simulink model "ARDroneWPTracking"  (R2018b)
settings: Solver=ode1  StartTime=0.0  StopTime=inf  FixedStep=sampleTime  RelTol=1e-3  EnableMultiTasking=on
undefined symbols (not defined in the file): Gxd_A_obs, Gxd_B_obs, Gxd_C_obs, Gyawd_A_obs, Gyawd_B_obs, Gyawd_C_obs, Gyd_A_obs, Gyd_B_obs, Gyd_C_obs, Gzd_A_obs, Gzd_B_obs, Gzd_C_obs, K0_X, K0_Y, K0_yaw, K0_Z, K_X, K_Y, K_yaw, K_Z, KGe_X, KGe_Y, KGe_yaw, KGe_Z, sampleTime, Standard_Devices, t_samp, UDP_Protocol, waypoints
libraries: sldrtlib x2, rtwinlib x1
CloseFcn:
  | rtwprivate ssgencode ModelCloseRequest Good_NL_model
settings Model: SimulationMode=external  ExtModeTrigDuration=100000  Creator=Paul  LastModifiedBy=Henrique
settings DataIOCC: LimitDataPoints=on  SaveFormat=Array  SignalLoggingSaveFormat=ModelDataLogs  TimeSaveName=time
settings OptimizationCC: ExpressionDepthLimit=2147483647  InitFltsAndDblsToZero=on
settings DebuggingCC: UnderspecifiedInitializationDetection=Classic  MergeDetectMultiDrivingBlocksExec=none  SolverPrmCheckMsg=warning  FcnCallInpInsideContextMsg=warning  StateNameClashWarn=warning  SFUnexpectedBacktrackingDiag=warning  SFNoUnconditionalDefaultTransitionDiag=warning  SFExecutionAtInitializationDiag=none
settings ModelReferenceCC: PropagateSignalLabelsOutOfModel=off
settings SFSimCC: SimUseLocalCustomCode=off
settings RTWCC: SystemTargetFile=sldrt.tlc  TemplateMakefile=sldrt.tmf  Description=Simulink Desktop Real-Time  RTWUseLocalCustomCode=off  RTWCompilerOptimization=on
settings CodeAppCC: MaxIdLength=95  StateflowObjectComments=on
settings SimulinkDesktopRealTimeCC: TargetPreCompLibLocation=D:\Programas\MATLAB 2018b\toolbox\sldrt\lib\win64  TargetLangStandard=C89/C90 (ANSI)  SupportVariableSizeSignals=off  PreserveStateflowLocalDataDimensions=off
settings ConfigComp: CovMetricSettings=dw  CovHtmlReporting=on  CovSaveCumulativeToWorkspaceVar=on  CovSaveSingleToWorkspaceVar=on  CovExternalEMLEnable=off

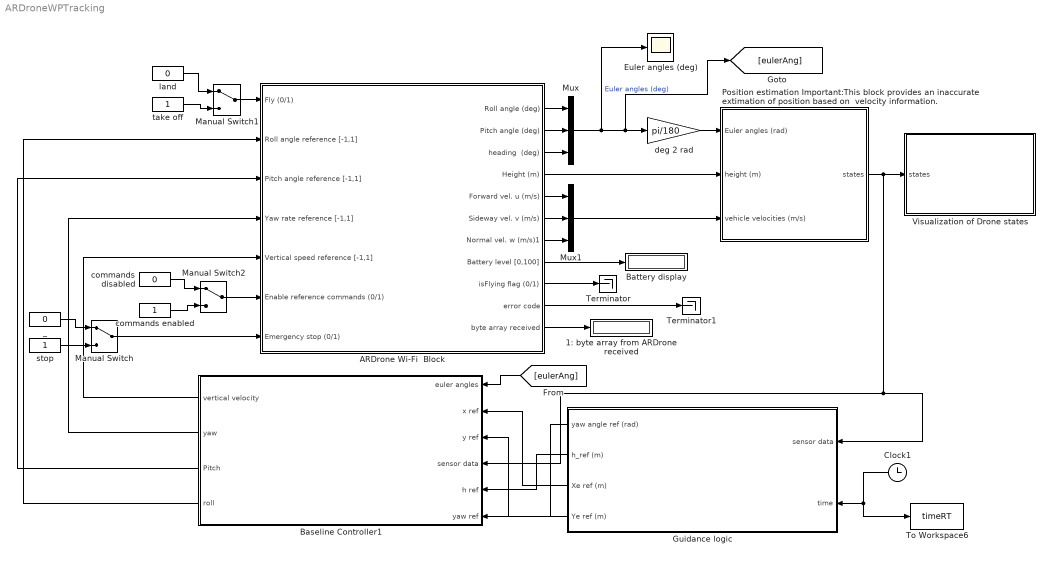
== system ARDroneWPTracking ==
  "1: byte array from ARDrone received " : Display
  ARDrone Wi-Fi  Block : Subsystem  AncestorBlock="ARBlocks/ARDrone Wi-Fi  Block"
  Baseline Controller1 : Subsystem  AncestorBlock=ARBlocks/Baseline Controller
  Battery display : Display
  Clock1 : Clock
  Euler angles (deg) : Scope
  Guidance logic : Subsystem  AncestorBlock=ARBlocks/Guidance logic
  Manual Switch : ManualSwitch
  Manual Switch1 : ManualSwitch
  Manual Switch2 : ManualSwitch
  Mux : Mux  Inputs=3
  Mux1 : Mux  Inputs=3
  "Position estimation Important:This block provides an inaccurate extimation of position based on  velocity information. " : Subsystem  AncestorBlock=|
      | ARBlocks/Position estimation
      | Important:This block provides an 
      | inaccurate extimation of position 
      | based on  velocity information.
  Terminator : Terminator
  Terminator1 : Terminator
  To Workspace6 : ToWorkspace  VariableName=timeRT  SampleTime=sampleTime
  Visualization of Drone states : Subsystem
  _ : Constant  Value=0
  commands disabled : Constant  Value=0
  commands enabled : Constant
  deg 2 rad : Gain  Gain=pi/180
  land : Constant  Value=0
  stop : Constant
  take off : Constant
  wires:
  _/1 -> Manual Switch/1
  stop/1 -> Manual Switch/2
  land/1 -> Manual Switch1/1
  take off/1 -> Manual Switch1/2
  commands disabled/1 -> Manual Switch2/1
  commands enabled/1 -> Manual Switch2/2
  Manual Switch1/1 -> ARDrone Wi-Fi  Block/1(Fly (0/1))
  Manual Switch2/1 -> ARDrone Wi-Fi  Block/6(Enable reference commands (0/1))
  Manual Switch/1 -> ARDrone Wi-Fi  Block/7(Emergency stop (0/1))
  ARDrone Wi-Fi  Block/1(Roll angle (deg)) -> Mux/1
  ARDrone Wi-Fi  Block/2(Pitch angle (deg)) -> Mux/2
  ARDrone Wi-Fi  Block/5(Forward vel. u (m/s)) -> Mux1/1
  ARDrone Wi-Fi  Block/6(Sideway vel. v (m/s)) -> Mux1/2
  ARDrone Wi-Fi  Block/7(Normal vel. w (m/s)1) -> Mux1/3
  Mux/1 -> Euler angles (deg)/1, [eulerAng], deg 2 rad/1  "Euler angles (deg)"
  ARDrone Wi-Fi  Block/8(Battery level [0,100]) -> Battery display/1
  "Position estimation Important:This block provides an inaccurate extimation of position based on  velocity information. "/1(states) -> Baseline Controller1/4(sensor data), Guidance logic/1(sensor data), Visualization of Drone states/1(states)
  deg 2 rad/1 -> "Position estimation Important:This block provides an inaccurate extimation of position based on  velocity information. "/1(Euler angles (rad))
  ARDrone Wi-Fi  Block/4(Height (m)) -> "Position estimation Important:This block provides an inaccurate extimation of position based on  velocity information. "/2(height (m))
  Mux1/1 -> "Position estimation Important:This block provides an inaccurate extimation of position based on  velocity information. "/3(vehicle velocities (m/s))
  Clock1/1 -> To Workspace6/1, Guidance logic/2(time)
  ARDrone Wi-Fi  Block/3(heading  (deg)) -> Mux/3
  Guidance logic/2(h_ref (m)) -> Baseline Controller1/5(h ref)
  Guidance logic/4(Ye ref (m)) -> Baseline Controller1/3(y ref)
  Guidance logic/1(yaw angle ref (rad)) -> Baseline Controller1/6(yaw ref)
  ARDrone Wi-Fi  Block/9(isFlying flag (0/1)) -> Terminator/1
  ARDrone Wi-Fi  Block/10(error code) -> Terminator1/1
  ARDrone Wi-Fi  Block/11(byte array received) -> "1: byte array from ARDrone received "/1
  Guidance logic/3(Xe ref (m)) -> Baseline Controller1/2(x ref)
  [eulerAng] -> Baseline Controller1/1(euler angles)
  Baseline Controller1/1("vertical velocity ") -> ARDrone Wi-Fi  Block/5(Vertical speed reference [-1,1])
  Baseline Controller1/2("yaw ") -> ARDrone Wi-Fi  Block/4(Yaw rate reference [-1,1])
  Baseline Controller1/3("Pitch ") -> ARDrone Wi-Fi  Block/3(Pitch angle reference [-1,1])
  Baseline Controller1/4("roll ") -> ARDrone Wi-Fi  Block/2(Roll angle reference [-1,1])

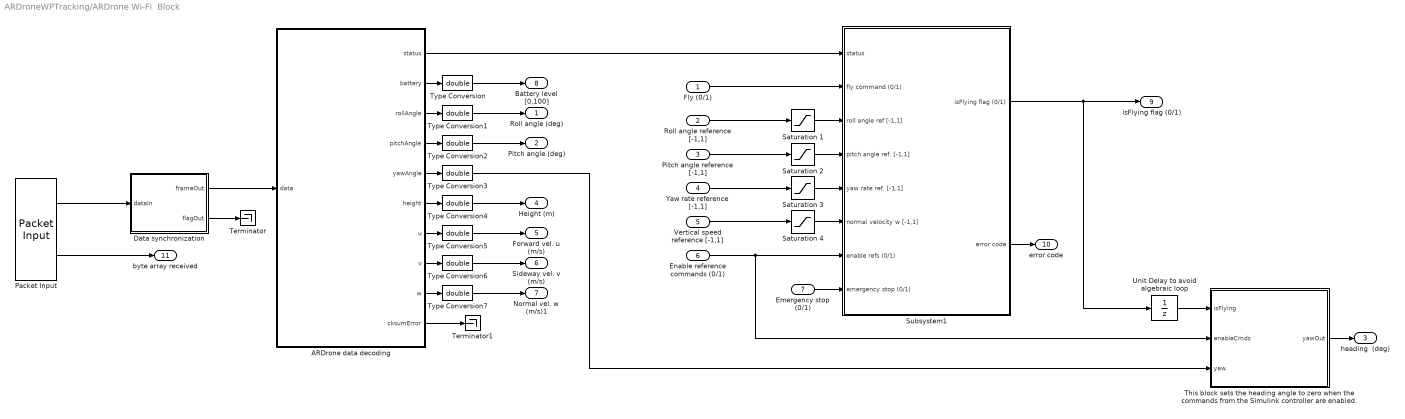
== system ARDroneWPTracking/ARDrone Wi-Fi  Block ==
  Fly (0/1) : Inport
  Roll angle reference [-1,1] : Inport  Port=2
  Pitch angle reference [-1,1] : Inport  Port=3
  Yaw rate reference [-1,1] : Inport  Port=4
  Vertical speed reference [-1,1] : Inport  Port=5
  Enable reference commands (0/1) : Inport  Port=6
  Emergency stop (0/1) : Inport  Port=7
  ARDrone data decoding : MATLAB Function  TreatAsAtomicUnit=on
  "Data synchronization " : MATLAB Function  TreatAsAtomicUnit=on
  Packet Input : sldrtlib/Packet Input  SampleTime=sampleTime  MaxMissedTicks=1  ShowMissedTicks=off  YieldWhenWaiting=off  DrvName=Standard_Devices/UDP_Protocol  DrvAddress=5554  DrvOptions=[3232235777 5554]  PacketSize=500  DataTypes='500*uint8'  ShowReady=on  ShowError=off  PacketID=1  ByteOrder=1  ShowTimestamp=off
      settings: AttributesFormatString=Standard Devices\nUDP Protocol [15B2h]  SourceProductName=Simulink Desktop Real-Time
  Saturation {1..4} (4 alike) : Saturate  UpperLimit=1  LowerLimit=-1
  Subsystem1 : Subsystem
  Terminator : Terminator
  Terminator1 : Terminator
  "This block sets the heading angle to zero when the commands from the Simulink controller are enabled. " : MATLAB Function  TreatAsAtomicUnit=on
  Type Conversion{,1..7} (8 alike) : DataTypeConversion  OutDataTypeStr=double
  Unit Delay to avoid algebraic loop : UnitDelay  SampleTime=-1
  Roll angle (deg) : Outport
  Pitch angle (deg) : Outport  Port=2
  heading  (deg) : Outport  Port=3
  Height (m) : Outport  Port=4
  Forward vel. u (m/s) : Outport  Port=5
  Sideway vel. v (m/s) : Outport  Port=6
  Normal vel. w (m/s)1 : Outport  Port=7
  Battery level [0,100] : Outport  Port=8
  isFlying flag (0/1) : Outport  Port=9
  error code : Outport  Port=10
  byte array received : Outport  Port=11
  wires:
  Unit Delay to avoid algebraic loop/1 -> "This block sets the heading angle to zero when the commands from the Simulink controller are enabled. "/1(isFlying)
  "Data synchronization "/2(flagOut) -> Terminator/1
  Saturation 4/1 -> Subsystem1/6(normal velocity w [-1,1])
  Saturation 3/1 -> Subsystem1/5(yaw rate ref. [-1,1])
  Saturation 2/1 -> Subsystem1/4(pitch angle ref. [-1,1])
  Saturation 1/1 -> Subsystem1/3(roll angle ref [-1,1])
  Fly (0/1)/1 -> Subsystem1/2(fly command (0/1))
  "This block sets the heading angle to zero when the commands from the Simulink controller are enabled. "/1(yawOut) -> heading  (deg)/1
  Type Conversion3/1 -> "This block sets the heading angle to zero when the commands from the Simulink controller are enabled. "/3(yaw)
  Type Conversion7/1 -> Normal vel. w (m/s)1/1
  Type Conversion6/1 -> Sideway vel. v (m/s)/1
  Type Conversion5/1 -> Forward vel. u (m/s)/1
  Type Conversion4/1 -> Height (m)/1
  Type Conversion2/1 -> Pitch angle (deg)/1
  Type Conversion1/1 -> Roll angle (deg)/1
  Type Conversion/1 -> Battery level [0,100]/1
  ARDrone data decoding/10(cksumError) -> Terminator1/1
  Subsystem1/2(error code) -> error code/1
  Subsystem1/1(isFlying flag (0/1)) -> Unit Delay to avoid algebraic loop/1, isFlying flag (0/1)/1
  Emergency stop (0/1)/1 -> Subsystem1/8(emergency stop (0/1))
  Enable reference commands (0/1)/1 -> Subsystem1/7(enable refs (0/1)), "This block sets the heading angle to zero when the commands from the Simulink controller are enabled. "/2(enableCmds)
  Vertical speed reference [-1,1]/1 -> Saturation 4/1
  Yaw rate reference [-1,1]/1 -> Saturation 3/1
  Pitch angle reference [-1,1]/1 -> Saturation 2/1
  Roll angle reference [-1,1]/1 -> Saturation 1/1
  ARDrone data decoding/1(status) -> Subsystem1/1(status)
  Packet Input/2 -> byte array received/1
  ARDrone data decoding/9(w) -> Type Conversion7/1
  ARDrone data decoding/8(v) -> Type Conversion6/1
  ARDrone data decoding/7(u) -> Type Conversion5/1
  ARDrone data decoding/4(pitchAngle) -> Type Conversion2/1
  ARDrone data decoding/3(rollAngle) -> Type Conversion1/1
  ARDrone data decoding/6(height) -> Type Conversion4/1
  ARDrone data decoding/2(battery) -> Type Conversion/1
  ARDrone data decoding/5(yawAngle) -> Type Conversion3/1
  "Data synchronization "/1(frameOut) -> ARDrone data decoding/1(data)
  Packet Input/1 -> "Data synchronization "/1(dataIn)

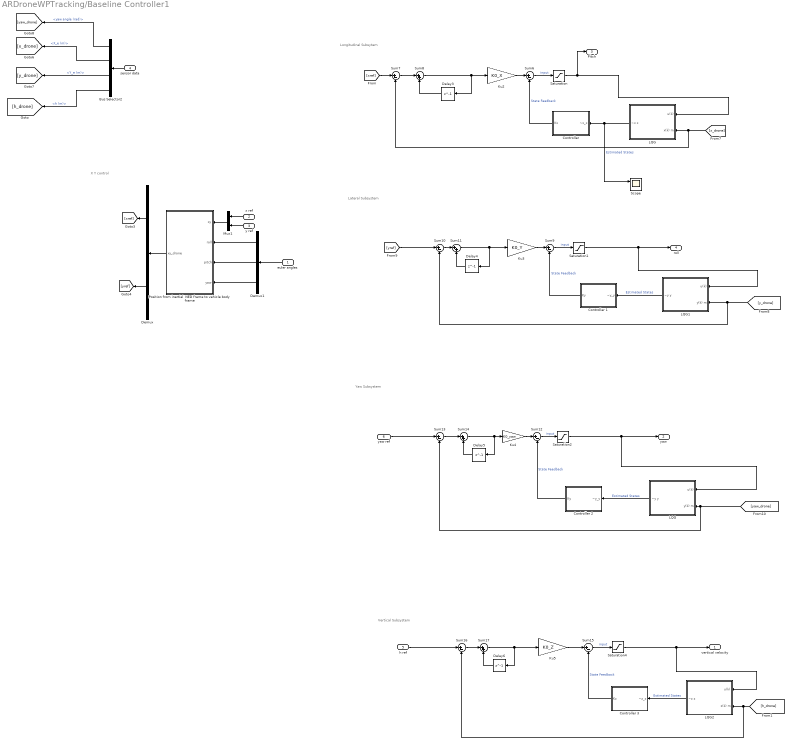
== system ARDroneWPTracking/Baseline Controller1 ==
  note: Vertical Subsystem
  note: X Y control
  note: Yaw Subsystem
  note: Lateral Subsystem
  note: Longitudinal Subsytem
  euler angles : Inport
  x ref : Inport  Port=2
  y ref : Inport  Port=3
  sensor data : Inport  Port=4
  h ref : Inport  Port=5
  yaw ref : Inport  Port=6
  Bus Selector2 : BusSelector  OutputSignals=yaw angle (rad),X_e (m),Y_e (m),h (m)
  "Controller " : Subsystem
  Controller 1 : Subsystem
  Controller 2 : Subsystem
  Controller 3 : Subsystem
  Delay{3..6} (4 alike) : Delay  DelayLength=1  InitialCondition=0
  Demux : Demux  Outputs=2
  Demux1 : Demux  Outputs=3
  Ku2 : Gain  Gain=K0_X
  Ku3 : Gain  Gain=K0_Y
  Ku4 : Gain  Gain=K0_yaw
  Ku5 : Gain  Gain=K0_Z
  LQG : Subsystem
  "LQG " : Subsystem
  LQG1 : Subsystem
  LQG2 : Subsystem
  Mux1 : Mux  Inputs=2
  Position from inertial  NED frame to vehicle body frame : MATLAB Function  TreatAsAtomicUnit=on
  Saturation : Saturate  UpperLimit=2  LowerLimit=-1.2
  Saturation1 : Saturate  UpperLimit=1.2  LowerLimit=-1.2
  Saturation2 : Saturate  UpperLimit=1.2  LowerLimit=-1.2
  Saturation4 : Saturate  UpperLimit=1.2  LowerLimit=-1.2
  Scope : Scope  NumInputPorts=2
  Sum{6..7,9..10,12..13,15..16} (8 alike) : Sum  Inputs=|+-
  Sum{8,11,14,17} (4 alike) : Sum  Inputs=|++
  "vertical velocity " : Outport
  "yaw " : Outport  Port=2
  "Pitch " : Outport  Port=3
  "roll " : Outport  Port=4
  wires:
  LQG/1("~x x ") -> Scope/1, "Controller "/1(~x_x)  "Estimated States"
  Sum17/1 -> Ku5/1, Delay6/1
  Controller 3/1(Kz) -> Sum15/2  "State Feedback"
  Demux/2 -> [yref]
  [h_drone] -> Sum16/2, LQG2/2(z(k) m)
  Saturation1/1 -> "roll "/1, LQG1/1(u(k))
  Ku4/1 -> Sum12/1
  Saturation4/1 -> "vertical velocity "/1, LQG2/1(u(k))
  [yref] -> Sum10/1
  Sum11/1 -> Delay4/1, Ku3/1
  LQG2/1("~z z ") -> Controller 3/1(~z_z)  "Estimated States"
  Ku5/1 -> Sum15/1
  Sum10/1 -> Sum11/1
  "LQG "/1("~y y ") -> Controller 2/1(~y_y)  "Estimated States"
  Controller 2/1(Ky) -> Sum12/2  "State Feedback"
  Saturation2/1 -> "yaw "/1, "LQG "/1(u(k))
  Sum12/1 -> Saturation2/1  "input"
  "Controller "/1(Kx) -> Sum6/2  "State Feedback"
  yaw ref/1 -> Sum13/1
  euler angles/1 -> Demux1/1
  LQG1/1("~y y ") -> Controller 1/1(~y_y)  "Estimated States"
  [yaw_drone] -> Sum13/2, "LQG "/2(y(k) m)
  Sum16/1 -> Sum17/1
  Sum13/1 -> Sum14/1
  Sum15/1 -> Saturation4/1  "input"
  Sum8/1 -> Ku2/1, Delay3/1
  Delay5/1 -> Sum14/2
  [xref] -> Sum7/1
  Delay6/1 -> Sum17/2
  Mux1/1 -> Position from inertial  NED frame to vehicle body frame/1(xy)
  Demux/1 -> [xref]
  Demux1/1 -> Position from inertial  NED frame to vehicle body frame/2(roll)
  Delay4/1 -> Sum11/2
  Sum9/1 -> Saturation1/1  "input"
  [y_drone] -> Sum10/2, LQG1/2(y(k) m)
  Controller 1/1(Ky) -> Sum9/2  "State Feedback"
  h ref/1 -> Sum16/1
  Ku3/1 -> Sum9/1
  Sum14/1 -> Delay5/1, Ku4/1
  Demux1/2 -> Position from inertial  NED frame to vehicle body frame/3(pitch)
  Bus Selector2/4 -> [h_drone]  "<h (m)>"
  Sum7/1 -> Sum8/1
  Delay3/1 -> Sum8/2
  Demux1/3 -> Position from inertial  NED frame to vehicle body frame/4(yaw)
  Ku2/1 -> Sum6/1
  Bus Selector2/1 -> [yaw_drone]  "<yaw angle (rad)>"
  Saturation/1 -> "Pitch "/1, LQG/1(u(k))
  y ref/1 -> Mux1/2
  sensor data/1 -> Bus Selector2/1
  Bus Selector2/2 -> [x_drone]  "<X_e (m)>"
  Position from inertial  NED frame to vehicle body frame/1(xy_drone) -> Demux/1
  Bus Selector2/3 -> [y_drone]  "<Y_e (m)>"
  x ref/1 -> Mux1/1
  Sum6/1 -> Saturation/1  "input"
  [x_drone] -> Sum7/2, LQG/2(x(k) m)

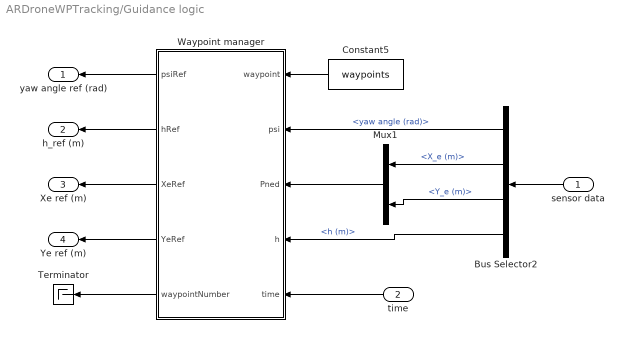
== system ARDroneWPTracking/Guidance logic ==
  sensor data : Inport
  time : Inport  Port=2
  Bus Selector2 : BusSelector  OutputSignals=yaw angle (rad),X_e (m),Y_e (m),h (m)
  Constant5 : Constant  Value=waypoints  VectorParams1D=off
  Mux1 : Mux  Inputs=2
  Terminator : Terminator
  "Waypoint manager " : MATLAB Function  TreatAsAtomicUnit=on
  yaw angle ref (rad) : Outport
  h_ref (m) : Outport  Port=2
  Xe ref (m) : Outport  Port=3
  Ye ref (m) : Outport  Port=4
  wires:
  Constant5/1 -> "Waypoint manager "/1(waypoint)
  "Waypoint manager "/1(psiRef) -> yaw angle ref (rad)/1
  "Waypoint manager "/5(waypointNumber) -> Terminator/1
  time/1 -> "Waypoint manager "/5(time)
  Bus Selector2/4 -> "Waypoint manager "/4(h)  "<h (m)>"
  "Waypoint manager "/4(YeRef) -> Ye ref (m)/1
  "Waypoint manager "/3(XeRef) -> Xe ref (m)/1
  "Waypoint manager "/2(hRef) -> h_ref (m)/1
  Mux1/1 -> "Waypoint manager "/3(Pned)
  Bus Selector2/1 -> "Waypoint manager "/2(psi)  "<yaw angle (rad)>"
  sensor data/1 -> Bus Selector2/1
  Bus Selector2/3 -> Mux1/2  "<Y_e (m)>"
  Bus Selector2/2 -> Mux1/1  "<X_e (m)>"

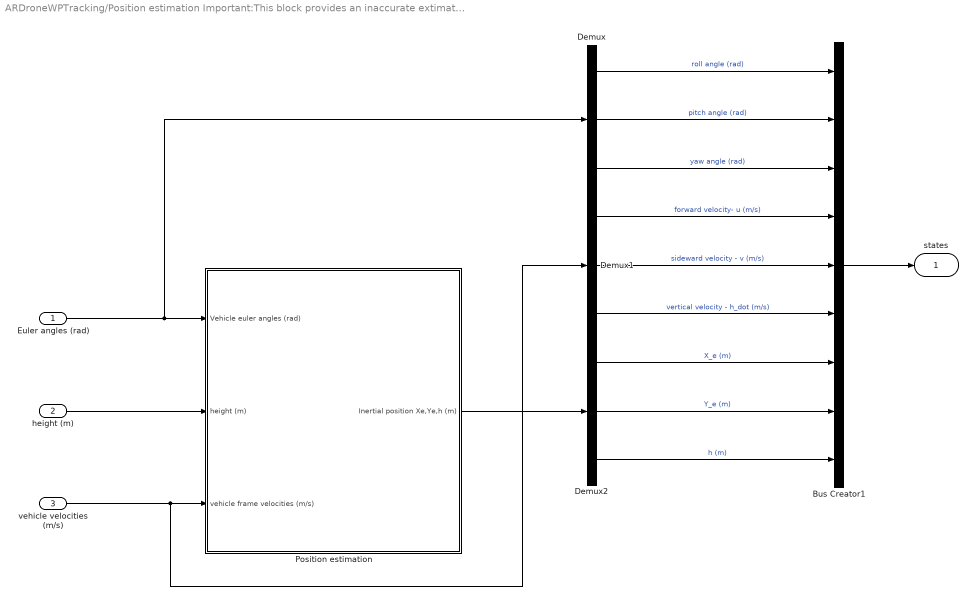
== system ARDroneWPTracking/Position estimation Important:This block provides an inaccurate extimation of position based on  velocity information.  ==
  Euler angles (rad) : Inport
  height (m) : Inport  Port=2
  vehicle velocities (m/s) : Inport  Port=3
  Bus Creator1 : BusCreator  Inputs=9
  Demux : Demux  Outputs=3
  Demux1 : Demux  Outputs=3
  Demux2 : Demux  Outputs=3
  Position estimation : Subsystem
  states : Outport
  wires:
  height (m)/1 -> Position estimation/2(height (m))
  Bus Creator1/1 -> states/1
  Demux2/3 -> Bus Creator1/9  "h (m)"
  Demux2/2 -> Bus Creator1/8  "Y_e (m)"
  Demux2/1 -> Bus Creator1/7  "X_e (m)"
  Demux1/3 -> Bus Creator1/6  "vertical velocity - h_dot (m/s)"
  Demux1/2 -> Bus Creator1/5  "sideward velocity - v (m/s)"
  Demux1/1 -> Bus Creator1/4  "forward velocity- u (m/s)"
  Demux/3 -> Bus Creator1/3  "yaw angle (rad)"
  Demux/2 -> Bus Creator1/2  "pitch angle (rad)"
  Demux/1 -> Bus Creator1/1  "roll angle (rad)"
  Position estimation/1(Inertial position Xe,Ye,h (m)) -> Demux2/1
  Euler angles (rad)/1 -> Demux/1, Position estimation/1(Vehicle euler angles (rad))
  vehicle velocities (m/s)/1 -> Position estimation/3(vehicle frame velocities (m/s)), Demux1/1

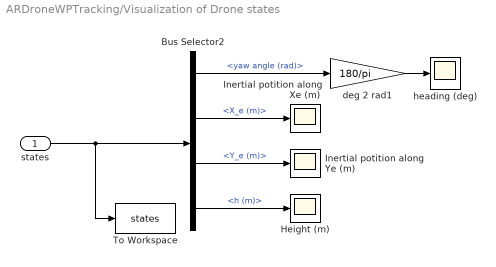
== system ARDroneWPTracking/Visualization of Drone states ==
  states : Inport
  Bus Selector2 : BusSelector  OutputSignals=yaw angle (rad),X_e (m),Y_e (m),h (m)
  Height (m) : Scope
  Inertial potition along Xe (m) : Scope
  Inertial potition along Ye (m) : Scope
  To Workspace : ToWorkspace  VariableName=states  SaveFormat=Structure With Time  SampleTime=-1
  deg 2 rad1 : Gain  Gain=180/pi
  heading (deg) : Scope
  wires:
  states/1 -> To Workspace/1, Bus Selector2/1
  Bus Selector2/1 -> deg 2 rad1/1  "<yaw angle (rad)>"
  Bus Selector2/2 -> Inertial potition along Xe (m)/1  "<X_e (m)>"
  Bus Selector2/3 -> Inertial potition along Ye (m)/1  "<Y_e (m)>"
  Bus Selector2/4 -> Height (m)/1  "<h (m)>"
  deg 2 rad1/1 -> heading (deg)/1

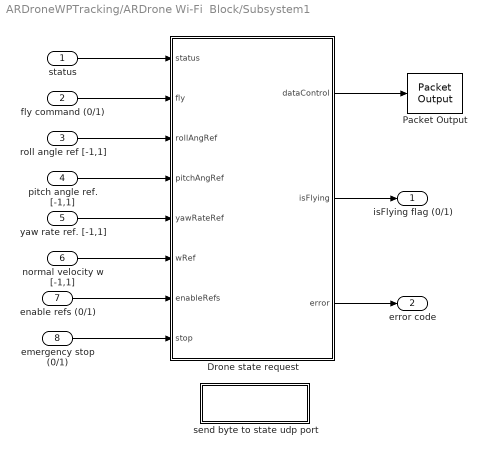
== system ARDroneWPTracking/ARDrone Wi-Fi  Block/Subsystem1 ==
  status : Inport
  fly command (0/1) : Inport  Port=2
  roll angle ref [-1,1] : Inport  Port=3
  pitch angle ref. [-1,1] : Inport  Port=4
  yaw rate ref. [-1,1] : Inport  Port=5
  normal velocity w [-1,1] : Inport  Port=6
  enable refs (0/1) : Inport  Port=7
  emergency stop (0/1) : Inport  Port=8
  Drone state request : MATLAB Function  TreatAsAtomicUnit=on
  Packet Output : sldrtlib/Packet Output  SampleTime=-1  MaxMissedTicks=10  ShowMissedTicks=off  YieldWhenWaiting=off  DrvName=Standard_Devices/UDP_Protocol  DrvAddress=5556  DrvOptions=[3232235777 5556]  PacketSize=150  DataTypes='150*uint8'  ShowReady=off  ShowError=off  PacketID=1  ByteOrder=1  InitialValue=[]  FinalValue=[]
      settings: AttributesFormatString=Standard Devices\nUDP Protocol [15B4h]  SourceProductName=Simulink Desktop Real-Time
  "send byte to state udp port " : Subsystem
  isFlying flag (0/1) : Outport
  error code : Outport  Port=2
  wires:
  Drone state request/3(error) -> error code/1
  emergency stop (0/1)/1 -> Drone state request/8(stop)
  enable refs (0/1)/1 -> Drone state request/7(enableRefs)
  normal velocity w [-1,1]/1 -> Drone state request/6(wRef)
  yaw rate ref. [-1,1]/1 -> Drone state request/5(yawRateRef)
  roll angle ref [-1,1]/1 -> Drone state request/3(rollAngRef)
  Drone state request/2(isFlying) -> isFlying flag (0/1)/1
  Drone state request/1(dataControl) -> Packet Output/1
  status/1 -> Drone state request/1(status)
  pitch angle ref. [-1,1]/1 -> Drone state request/4(pitchAngRef)
  fly command (0/1)/1 -> Drone state request/2(fly)

== system ARDroneWPTracking/Baseline Controller1/Controller  ==
  ~x_x : Inport
  "LQR Gain " : Gain  Gain=K_X  Multiplication=Matrix(K*u) (u vector)
  Kx : Outport
  wires:
  ~x_x/1 -> "LQR Gain "/1
  "LQR Gain "/1 -> Kx/1

== system ARDroneWPTracking/Baseline Controller1/Controller 1 ==
  ~y_y : Inport
  Gain : Gain  Gain=K_Y  Multiplication=Matrix(K*u) (u vector)
  Ky : Outport
  wires:
  ~y_y/1 -> Gain/1
  Gain/1 -> Ky/1

== system ARDroneWPTracking/Baseline Controller1/Controller 2 ==
  ~y_y : Inport
  Gain : Gain  Gain=K_yaw  Multiplication=Matrix(K*u) (u vector)
  Ky : Outport
  wires:
  ~y_y/1 -> Gain/1
  Gain/1 -> Ky/1

== system ARDroneWPTracking/Baseline Controller1/Controller 3 ==
  ~z_z : Inport
  Gain : Gain  Gain=K_Z  Multiplication=Matrix(K*u) (u vector)
  Kz : Outport
  wires:
  ~z_z/1 -> Gain/1
  Gain/1 -> Kz/1

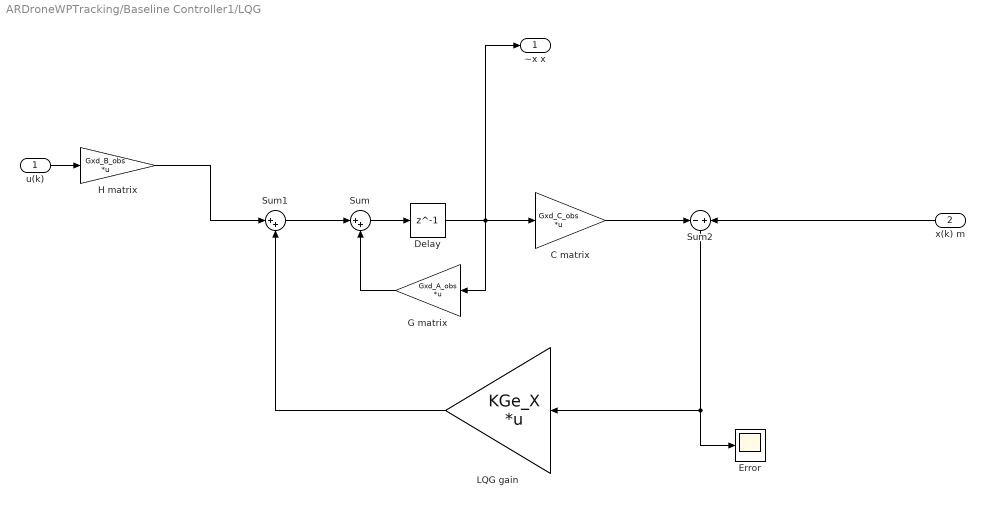
== system ARDroneWPTracking/Baseline Controller1/LQG ==
  u(k) : Inport
  x(k) m : Inport  Port=2
  C matrix : Gain  Gain=Gxd_C_obs  Multiplication=Matrix(K*u)
  Delay : Delay  DelayLength=1  InitialCondition=0  SampleTime=t_samp
  Error : Scope
  G matrix : Gain  Gain=Gxd_A_obs  Multiplication=Matrix(K*u)
  H matrix : Gain  Gain=Gxd_B_obs  Multiplication=Matrix(K*u)
  LQG gain : Gain  Gain=KGe_X  Multiplication=Matrix(K*u)
  Sum : Sum  Inputs=|++
  Sum1 : Sum  Inputs=|++
  Sum2 : Sum  Inputs=-+
  "~x x " : Outport
  wires:
  C matrix/1 -> Sum2/1
  x(k) m/1 -> Sum2/2
  H matrix/1 -> Sum1/1
  Sum/1 -> Delay/1
  u(k)/1 -> H matrix/1
  G matrix/1 -> Sum/2
  Sum2/1 -> Error/1, LQG gain/1
  LQG gain/1 -> Sum1/2
  Delay/1 -> "~x x "/1, G matrix/1, C matrix/1
  Sum1/1 -> Sum/1

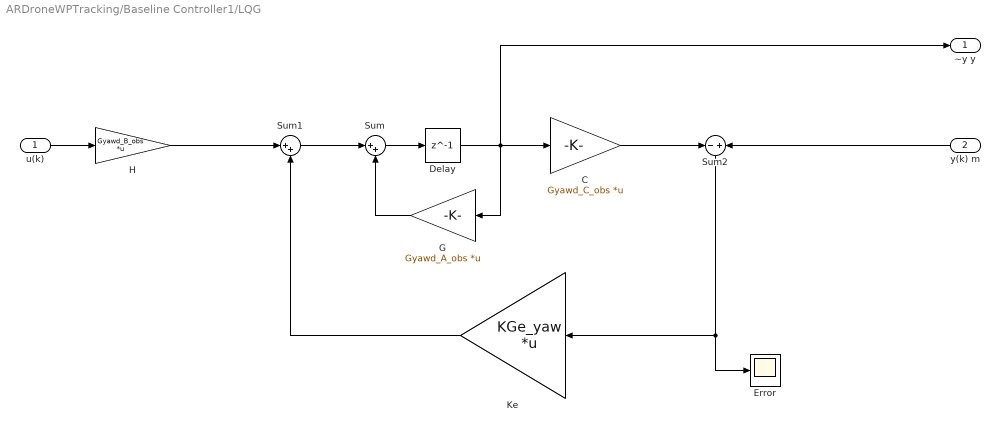
== system ARDroneWPTracking/Baseline Controller1/LQG  ==
  u(k) : Inport
  y(k) m : Inport  Port=2
  C : Gain  Gain=Gyawd_C_obs  Multiplication=Matrix(K*u)
  Delay : Delay  DelayLength=1  InitialCondition=0  SampleTime=t_samp
  Error : Scope
  G : Gain  Gain=Gyawd_A_obs  Multiplication=Matrix(K*u)
  H : Gain  Gain=Gyawd_B_obs  Multiplication=Matrix(K*u)
  Ke : Gain  Gain=KGe_yaw  Multiplication=Matrix(K*u)
  Sum : Sum  Inputs=|++
  Sum1 : Sum  Inputs=|++
  Sum2 : Sum  Inputs=-+
  "~y y " : Outport
  wires:
  C/1 -> Sum2/1
  y(k) m/1 -> Sum2/2
  H/1 -> Sum1/1
  Sum/1 -> Delay/1
  u(k)/1 -> H/1
  G/1 -> Sum/2
  Sum2/1 -> Error/1, Ke/1
  Sum1/1 -> Sum/1
  Ke/1 -> Sum1/2
  Delay/1 -> "~y y "/1, G/1, C/1

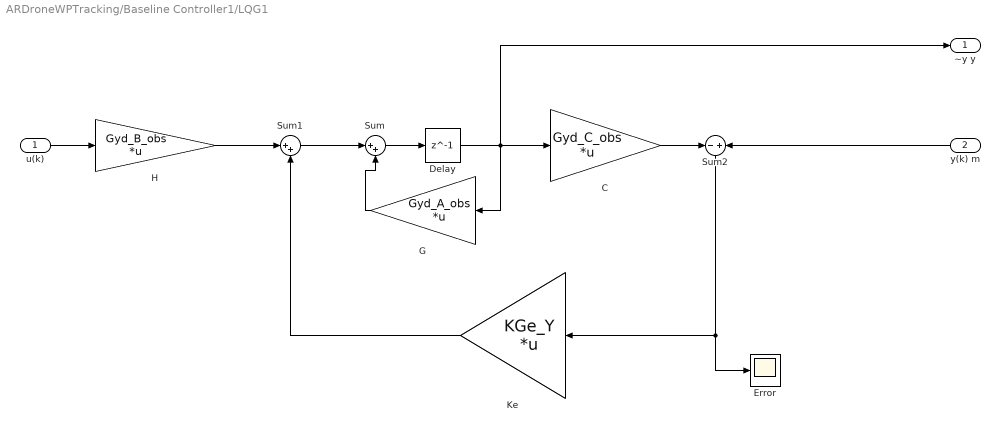
== system ARDroneWPTracking/Baseline Controller1/LQG1 ==
  u(k) : Inport
  y(k) m : Inport  Port=2
  C : Gain  Gain=Gyd_C_obs  Multiplication=Matrix(K*u)
  Delay : Delay  DelayLength=1  InitialCondition=0  SampleTime=t_samp
  Error : Scope
  G : Gain  Gain=Gyd_A_obs  Multiplication=Matrix(K*u)
  H : Gain  Gain=Gyd_B_obs  Multiplication=Matrix(K*u)
  Ke : Gain  Gain=KGe_Y  Multiplication=Matrix(K*u)
  Sum : Sum  Inputs=|++
  Sum1 : Sum  Inputs=|++
  Sum2 : Sum  Inputs=-+
  "~y y " : Outport
  wires:
  C/1 -> Sum2/1
  y(k) m/1 -> Sum2/2
  H/1 -> Sum1/1
  Sum/1 -> Delay/1
  u(k)/1 -> H/1
  G/1 -> Sum/2
  Sum2/1 -> Error/1, Ke/1
  Sum1/1 -> Sum/1
  Ke/1 -> Sum1/2
  Delay/1 -> "~y y "/1, C/1, G/1

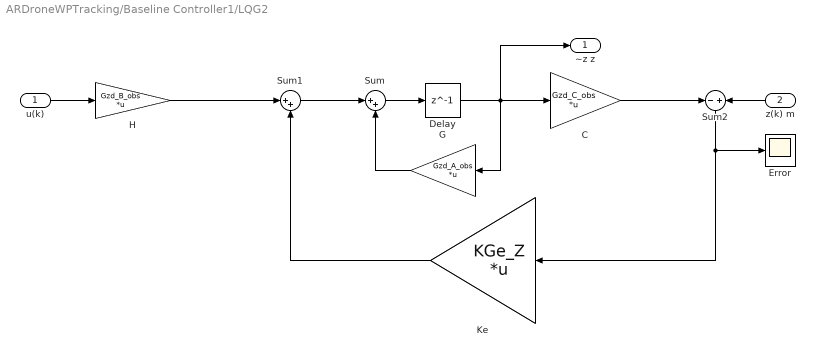
== system ARDroneWPTracking/Baseline Controller1/LQG2 ==
  u(k) : Inport
  z(k) m : Inport  Port=2
  C : Gain  Gain=Gzd_C_obs  Multiplication=Matrix(K*u)
  Delay : Delay  DelayLength=1  InitialCondition=0  SampleTime=t_samp
  Error : Scope
  G : Gain  Gain=Gzd_A_obs  Multiplication=Matrix(K*u)
  H : Gain  Gain=Gzd_B_obs  Multiplication=Matrix(K*u)
  Ke : Gain  Gain=KGe_Z  Multiplication=Matrix(K*u)
  Sum : Sum  Inputs=|++
  Sum1 : Sum  Inputs=|++
  Sum2 : Sum  Inputs=-+
  "~z z " : Outport
  wires:
  C/1 -> Sum2/1
  z(k) m/1 -> Sum2/2
  H/1 -> Sum1/1
  Sum/1 -> Delay/1
  u(k)/1 -> H/1
  G/1 -> Sum/2
  Sum2/1 -> Ke/1, Error/1
  Sum1/1 -> Sum/1
  Ke/1 -> Sum1/2
  Delay/1 -> G/1, "~z z "/1, C/1

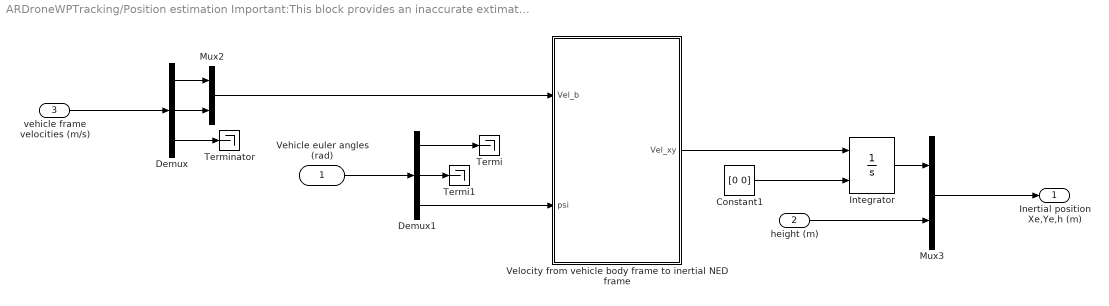
== system ARDroneWPTracking/Position estimation Important:This block provides an inaccurate extimation of position based on  velocity information. /Position estimation ==
  Vehicle euler angles (rad) : Inport
  height (m) : Inport  Port=2
  vehicle frame velocities (m/s) : Inport  Port=3
  Constant1 : Constant  Value=[0 0]
  Demux : Demux  Outputs=3
  Demux1 : Demux  Outputs=3
  Integrator : Integrator  InitialConditionSource=external
  Mux2 : Mux  Inputs=2
  Mux3 : Mux  Inputs=2
  Termi : Terminator
  Termi1 : Terminator
  Terminator : Terminator
  Velocity from vehicle body frame to inertial NED  frame : MATLAB Function  TreatAsAtomicUnit=on
  Inertial position Xe,Ye,h (m) : Outport
  wires:
  Mux3/1 -> Inertial position Xe,Ye,h (m)/1
  height (m)/1 -> Mux3/2
  Vehicle euler angles (rad)/1 -> Demux1/1
  vehicle frame velocities (m/s)/1 -> Demux/1
  Demux1/3 -> Velocity from vehicle body frame to inertial NED  frame/2(psi)
  Integrator/1 -> Mux3/1
  Constant1/1 -> Integrator/2
  Velocity from vehicle body frame to inertial NED  frame/1(Vel_xy) -> Integrator/1
  Demux1/2 -> Termi1/1
  Demux1/1 -> Termi/1
  Mux2/1 -> Velocity from vehicle body frame to inertial NED  frame/1(Vel_b)
  Demux/1 -> Mux2/1
  Demux/2 -> Mux2/2
  Demux/3 -> Terminator/1

== system ARDroneWPTracking/ARDrone Wi-Fi  Block/Subsystem1/send byte to state udp port  ==
  Constant : Constant  Value=[1 ;13]  OutDataTypeStr=uint8
  Packet Output1 : rtwinlib/Packet Output  SampleTime=sampleTime*10  MaxMissedTicks=10  ShowMissedTicks=off  YieldWhenWaiting=off  DrvName=Standard_Devices/UDP_Protocol  DrvAddress=5554  DrvOptions=[3232235777 5554]  PacketSize=2  DataTypes='2*uint8'  ShowReady=off  ShowError=off  PacketID=1  ByteOrder=1  InitialValue=[]  FinalValue=[]
      settings: AttributesFormatString=Standard Devices\nUDP Protocol [15B2h]  SourceProductName=Simulink Desktop Real-Time  SourceProductBaseCode=WT
  Rate Transition : RateTransition  OutPortSampleTime=sampleTime*10
  wires:
  Rate Transition/1 -> Packet Output1/1
  Constant/1 -> Rate Transition/1

== matlab function ARDroneWPTracking/ARDrone Wi-Fi  Block/Data synchronization  ==
  data: dataIn input; frameOut output; flagOut output
function [frameOut,flagOut]  = fcn(dataIn)
%#eml
%% Author: David Escobar Sanabria
%  Description: This function synchronizes data coming from the flight computer
%  computer. 
%  frameOut: Organized frame
%  frameIn: sequence of bytes not sync.
persistent frame; 
persistent lastFrame; 
persistent count; 
persistent countHeader; 
persistent countBuffer; 
persistent buffer; 

%% Size of byte array containing the data
sizePayload= 496;

%% Size of the array read each time step
nBytes = 500 ;%size(dataIn,1); 


%%%%%%%%%%%%%%%%%%%%%%%%%%%%%%%%%%%%%%%%%%%%%%%%%%%%%%%
%% Initialization of presistent variables
if isempty(buffer)
    buffer=uint8(zeros(1024,1));
end

if isempty(countBuffer)
    countBuffer=0;
end


if isempty(frame)
    frame=uint8(zeros(sizePayload,1));
end

if isempty(lastFrame)
    lastFrame=uint8(zeros(sizePayload,1));
end


if isempty(count)
    count=0;
end

if isempty(countHeader)
    countHeader=0;
end
%%%%%%%%%%%%%%%%%%%%%%%%%%%%%%%%%%%%%%%%%%%%%%%%%%%%%%%

%% Filling the buffer
buffer(countBuffer+1:countBuffer+nBytes) = dataIn;

bytesToRead = countBuffer+nBytes; 

%%%%%%%%%%%%%%%%%%%%%%%%%%%%%%%%%%%%%%%%%%%%%%%%%%%%%%%
%% Reading buffer

for k=1:bytesToRead    
    if(countHeader==4 && count<sizePayload)
        bytesLeft = sizePayload-count;
        frame(count+1:sizePayload) = buffer(k:k+bytesLeft-1);
        count = sizePayload;
        countBuffer = bytesToRead-bytesLeft ;
        buffer(1:countBuffer) = buffer(k+bytesLeft:bytesToRead);
        break;
        
    end
    
    if(countHeader==3 && buffer(k)==85)
        
        countHeader=4;
 
        if(bytesToRead-k > sizePayload)
            count =sizePayload;  
            frame(1:count) = buffer(k+1:k+sizePayload);  
            countBuffer =bytesToRead-k-sizePayload ; 
            buffer(1:countBuffer) = buffer(k+sizePayload+1:bytesToRead);
        else
            
            count =bytesToRead-k;
            if count > 0          
                frame(1:count) = buffer(k+1:bytesToRead);  
            end
            countBuffer = 0; 
            
        end
        
        break;
    end
    
    if(countHeader==2 && buffer(k)==102)
        countHeader=3;
    end
    
    if(countHeader==1 && buffer(k)==119)
        countHeader=2;
    end
       
    if(countHeader==0 && buffer(k)==136)
        countHeader=1;
    end

end

if count==sizePayload 
     frameOut = frame;
     flagOut = 1; 
     lastFrame = frame;
     frame=uint8(zeros(sizePayload,1));
     count=0;
     countHeader=0;
     
else % In case the buffer does not have an entire payload
    frameOut = lastFrame;
    flagOut = 0; 
end

== matlab function ARDroneWPTracking/ARDrone Wi-Fi  Block/ARDrone data decoding ==
  data: status output; battery output; rollAngle output; pitchAngle output; data input; yawAngle output; height output; u output; v output; w output; cksumError output
function [ status, battery,  rollAngle, pitchAngle, yawAngle, height, u,v,w , cksumError ]= fcn(data)
%#codegen

% Checksum array. cksum(1) contains the computed checksum, cksum(2)
% contains the checksum sent by the ARDrone. 
cksum = [0 0 ]; 

% Previous value of height 
persistent hPrev ; 
% Previous data packet
persistent dataPrev ; 

% Initialization of persistent variables
if isempty(hPrev)
    hPrev=0 ; 
end

if isempty(dataPrev)
    dataPrev = uint8(zeros(496,1)) ;
end

% Computing checksum
cksum(1) =  sum(double(data(1:end-8))) +442; 
% Checksum given by the drone
cksum(2) = double(data(end-3)) + double(data(end-2))*256 +  double(data(end-1))*256^2 + double(data(end))*256^3 ; 
% Checksum error
cksumError = abs(cksum(1)-cksum(2));
%% Change the following if statement to ensure that the data checksum is valid 
%if (data(15) == 148 && cksumError==0 )
if (data(15) == 148  )
    dataPrev = data; 
else
    data = dataPrev; 
end

% Converting bytes to drone information
status = getDroneState(data(1:4));
battery = decode(data(21:24),1); % unit: deg
pitchAngle = decode(data(25:28),0)/1000; % unit: deg
rollAngle = decode(data(29:32),0)/1000; % unit: deg
yawAngle = decode(data(33:36),0)/1000; % unit: deg
height = decode(data(37:40),1)/1000; % unit: deg
u = decode(data(41:44),0)/1000; % unit: m/s
v = decode(data(45:48),0)/1000; % unit: m/s
w = decode(data(49:52),0)/1000; % unit: m/s



if (status(32) ==1 && height< 0.2   )
    height = hPrev;
elseif status(32)==1 
    hPrev= height; 
end
  
    
end


function res = decode(input, mark)
% if mark = 1; then output a int
% else output the float value which is defined by SDK description.
% the input is an array (1*4) 
% e.g. : NDS(Battery_OS:Battery_OS+data_length-1)
    hex_value = dec2hex(input);
    hex_value = [hex_value(4,:),hex_value(3,:),hex_value(2,:),hex_value(1,:)];
    if mark ==1
        res = hex2dec(hex_value);
    else
        res = typecast(uint32(hex2dec(hex_value)),'single');
    end
end

function bin = getDroneState(input)
    bin = zeros(32,1); 
    hex = dec2hex(input);
    % put the hex_value in the order [31, 30......0]
    hex = [hex(4,:),hex(3,:),hex(2,:),hex(1,:)];
for i=1:length(hex)
    if hex(i)=='F'
        bin((i*4)-3:i*4)=[1 1 1 1];
    elseif hex(i)=='E'
        bin((i*4)-3:i*4)=[1 1 1 0];
    elseif hex(i)=='D'
        bin((i*4)-3:i*4)=[1 1 0 1];
    elseif hex(i)=='C'
        bin((i*4)-3:i*4)=[1 1 0 0];
    elseif hex(i)=='B'
        bin((i*4)-3:i*4)=[1 0 1 1];
    elseif hex(i)=='A'
        bin((i*4)-3:i*4)=[1 0 1 0];
    elseif hex(i)=='9'
        bin((i*4)-3:i*4)=[1 0 0 1];
    elseif hex(i)=='8'
        bin((i*4)-3:i*4)=[1 0 0 0];
    elseif hex(i)=='7'
        bin((i*4)-3:i*4)=[0 1 1 1];
    elseif hex(i)=='6'
        bin((i*4)-3:i*4)=[0 1 1 0];
    elseif hex(i)=='5'
        bin((i*4)-3:i*4)=[0 1 0 1];
    elseif hex(i)=='4'
        bin((i*4)-3:i*4)=[0 1 0 0];
    elseif hex(i)=='3'
        bin((i*4)-3:i*4)=[0 0 1 1];
    elseif hex(i)=='2'
        bin((i*4)-3:i*4)=[0 0 1 0];
    elseif hex(i)=='1'
        bin((i*4)-3:i*4)=[0 0 0 1];
    elseif hex(i)=='0'
        bin((i*4)-3:i*4)=[0 0 0 0];
    end
end

end

== matlab function ARDroneWPTracking/Baseline Controller1/Position from inertial  NED frame to vehicle body frame ==
  data: xy input; roll input; pitch input; yaw input; xy_drone output
function xy_drone = fcn(xy , roll, pitch, yaw)
%#codegen
T = [cos(yaw)*cos(pitch) (sin(roll)*sin(pitch)*cos(yaw) - cos(roll)*sin(yaw)); 
    cos(pitch)*sin(yaw) (sin(roll)*sin(pitch)*sin(yaw) + cos(roll)*cos(yaw))] ; 

xy_drone = (T')*xy(1:2,1);

== matlab function ARDroneWPTracking/ARDrone Wi-Fi  Block/Subsystem1/Drone state request ==
  data: status input; fly input; rollAngRef input; pitchAngRef input; yawRateRef input; wRef input; enableRefs input; dataControl output; isFlying output; stop input; error output
function [dataControl, isFlying, error] = fcn( status, fly, rollAngRef, pitchAngRef, yawRateRef, wRef, enableRefs, stop)
%#codegen

% Persistent variables.
persistent SequenceNumber ;

% Initialization of persistent variables at first time step. 

if isempty(SequenceNumber)
    SequenceNumber = 1 ;
end



% Error code / No error: 0
error=0;

% Boolean of flying status / Flying: 1
isFlying = status(32) ;

% Byte array of size 150 to be sent to the drone.
strOut = uint8(zeros(150,1)) ;

% String that coontains a variable size command. 
% cmd is concatenated with previous commands at each sample
cmd = '';

% At first time step and every 100 time steps, data is requested.
if (SequenceNumber <=1 || mod(SequenceNumber, 100) ==0 )
    SequenceNumber = SequenceNumber+1; 
    strCmd = getString(SequenceNumber) ;
    cmd = ['AT*CONFIG=' strCmd ',"general:navdata_demo","TRUE"' char(13)];
    
end

SequenceNumber = SequenceNumber+1;
strCmd = getString(SequenceNumber) ;
cmd = [cmd 'AT*COMWDG=' strCmd char(13)];


if stop ==1 % Emergency stop
   cmd = ['AT*REF=' strCmd ',290717952' char(13)] ; 
    
else % Not emergency stop
    
    if SequenceNumber >20 && SequenceNumber <22
        
        % Trim vehicle state estimation / angles set to zero
        SequenceNumber =SequenceNumber+1;
        strCmd = getString(SequenceNumber) ;
        cmd = [cmd 'AT*FTRIM=' strCmd char(13)] ;
        
    elseif SequenceNumber >=22 && SequenceNumber <25
        cmd = [cmd 'AT*CONFIG=' strCmd '"conrol:altitude_max","100000"' char(13)] ;
        
        
    elseif SequenceNumber >=25
        
        if ( fly == 1  )
            
            if (isFlying ==0)
                
                SequenceNumber =SequenceNumber+1;
                strCmd = getString(SequenceNumber) ;
                cmd = [cmd 'AT*REF=' strCmd ',290718208' char(13)] ;
            
            elseif isFlying==1 && enableRefs==1
                
                SequenceNumber =SequenceNumber+1;
                strCmd = getString(SequenceNumber) ;
                      
                cmd = [cmd 'AT*PCMD=' strCmd ',1,'] ;
                 
                aux = double (float2IEEE754 (rollAngRef) )  ;
                strAux = getString(abs(aux)) ; 
                if rollAngRef<0
                   strAux = [char(45) strAux] ; 
                end
                cmd = [cmd strAux ','];
                      
               aux = double (float2IEEE754 (pitchAngRef) ) ;
               strAux = getString(abs(aux)) ; 
               if pitchAngRef<0
                    strAux = [char(45) strAux] ; 
               end
               cmd = [cmd strAux ','];
                      
               aux =  double(float2IEEE754 (wRef)) ;
               strAux = getString(abs(aux)) ; 
               if wRef<0
                    strAux = [char(45) strAux] ; 
               end
               cmd = [cmd strAux ','];
                      
                      
               aux =  double (float2IEEE754 (yawRateRef) ) ;
               strAux = getString(abs(aux)) ; 
               if yawRateRef <0
                     error=2; 
                     strAux = [char(45) strAux] ; 
               end
               cmd = [cmd strAux char(13)];
               
                
            end
            
            
        elseif ( fly==0 )
                
               if isFlying ==1
                    SequenceNumber =SequenceNumber+1;
                    strCmd = getString(SequenceNumber) ;
                    cmd = [cmd 'AT*REF=' strCmd ',290717696' char(13)] ;
                    
               end
        end
        
    end
    
    
    
end

% cmd must contain less than 150 bytes. 
if (length(cmd)<150)
    strOut(1:length(cmd)) = cmd ;
else
    error =1; 
end

dataControl = strOut;

end


%% My str2num function that allows for code generation
function [ strOut] = getString( a )
d=1;

if (a<10)
    d=1;
end

if (a >=10 && a <100)
    d=2;
end

if (a >=100 && a <1000)
    d=3;
end

if (a >=1000 && a <10000)
    d=4;
end

if (a >=10000 && a <100000)
    d=5;
end

if (a >=100000 && a <1000000)
    d=6;
end

if (a >=1000000 && a <10000000)
    d=7;
end

if (a >=10000000 && a <100000000)
    d=8;
end

if (a >=100000000 && a <1000000000)
    d=9;
end

if (a >=1000000000 && a <10000000000)
    d=10;
end

if (a >=10000000000 )
    d=11;
end



digit = uint8(zeros(1,d)) ;
resTotal = 0;
%d = length(a) ;
for k=1:d
    
    res1 = mod(a,10^k)/(10^(k-1)) ;
    %( mod(a,10*k) - resTotal)/(10*k) ;
    
    digit(d-k+1) = char(48 + res1);
    resTotal = (10^(k-1))*res1 +resTotal;
    
end

strOut = char(digit) ;


end

%% Function to obtain a IEEE754 representation of a float number
function [ iVal ] = float2IEEE754( fVal )

binData = dec2bin(typecast (single(fVal), 'uint8'),8) 

binData2 =[ binData(4,:) binData(3,:) binData(2,:) binData(1,:)] 
iVal =0; 
for k=32:-1:1
    
    if (binData2(k) =='1')
        bit = 1;
    else
        bit =0;
    end
    
    if k == 1
        iVal = iVal - bit*2^(31);
    else
        iVal = iVal + bit*2^(32-k) ; 
    end
    
end

iVal = int32(iVal)

end

== matlab function ARDroneWPTracking/ARDrone Wi-Fi  Block/This block sets the heading angle to zero when the commands from the Simulink controller are enabled.  ==
  data: isFlying input; enableCmds input; yawOut output; yaw input
% Description: This function zeroes out the heading angle once the commands
% are enabled. 
function yawOut = fcn(isFlying,enableCmds,yaw)
%#codegen

yawOut = yaw; 
persistent yaw0 ; 
persistent mode ; 

if isempty (yaw0)
yaw0 = 0; 
end


if isempty (mode)
mode=0; 
end

if isFlying ==1 && enableCmds==1    
    yawOut = yaw - yaw0; 
    mode =1; 
elseif isFlying ==1 && mode ==0
    yaw0 = yaw; 
end


yawOut = mod(yawOut, 360) ;
if yawOut > 180
    yawOut = -360 + yawOut ; 
end

== matlab function ARDroneWPTracking/Position estimation Important:This block provides an inaccurate extimation of position based on  velocity information. /Position estimation/Velocity from vehicle body frame to inertial NED  frame ==
  data: Vel_b input; Vel_xy output; psi input
function Vel_xy = fcn(Vel_b , psi)
%#codegen
T = [cos(psi) -sin(psi) ; sin(psi) cos(psi)] ; 
Vel_xy = T*Vel_b;

== matlab function ARDroneWPTracking/Guidance logic/Waypoint manager  ==
  data: psiRef output; hRef output; waypoint input; psi input; Pned input; h input; XeRef output; YeRef output; time input; waypointNumber output
function [psiRef, hRef,  XeRef, YeRef, waypointNumber]       = fcn(waypoint, psi, Pned, h, time )
%#codegen

% Waypoint matrix contains final position, orientatoin, and waiting time.

% Number of waypoints
nPoints = size(waypoint, 2) ;

% Persitent variable used to keep trak of next waypoint
persistent wpointer;

% Time zero for each waypoint. This is used to wait at a desired position.
persistent t0 ;

% Init. persistent variables
if isempty(wpointer)
    wpointer = 1;
end

if isempty(t0)
    t0 = 0;
end

% A waypoint is reached if the distance between the desired waypoint and 
% the vehicle is less than 0.3 m in the XY plane, less than 0.3 m in height, 
% and less than 5 degrees in  heading. 

if ( norm(Pned(1:2,1) - waypoint(1:2, wpointer) )< 0.3 && ...
        norm(h - waypoint(3, wpointer)) < 0.3  && norm(psi - waypoint(4, wpointer) )< 5*pi/180   )
    
    if(wpointer ~= nPoints)
        
        if (t0 ==0)
            t0 = time;
        else
            if (time - t0 > waypoint(5, wpointer))
                
                 if(wpointer < nPoints)
                    wpointer = wpointer+ 1;
                    t0 = 0;
                 end
                
            end
        end
        
             
    end
    
       
    
end


%% Outputs:
hRef = waypoint(3, wpointer) ;
psiRef = waypoint(4, wpointer) ;
XeRef = waypoint(1, wpointer) ;
YeRef = waypoint(2, wpointer) ;
waypointNumber = wpointer ;
